simulink model "Filtro_pasa_bajo_2do_orden"  (R2023b)
settings: Solver=VariableStepAuto  StartTime=0.0  StopTime=10.0  RelTol=1e-3
undefined symbols (not defined in the file): wn, xita
settings Model: Creator=MSI  LastModifiedBy=MSI

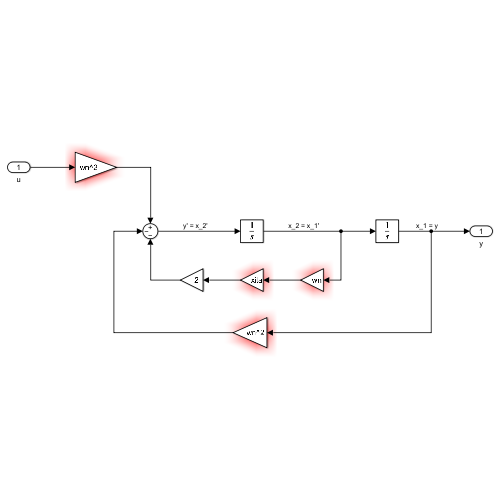
[thumbnail: Simulink's stored preview of the top-level diagram]
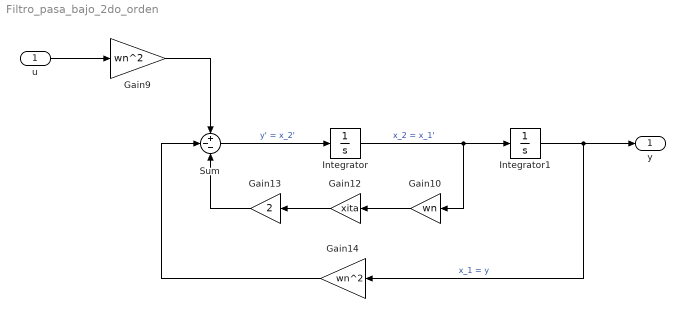
== system Filtro_pasa_bajo_2do_orden ==
  u : Inport
  Gain10 : Gain  Gain=wn
  Gain12 : Gain  Gain=xita
  Gain13 : Gain  Gain=2
  Gain14 : Gain  Gain=wn^2
  Gain9 : Gain  Gain=wn^2
  Integrator : Integrator
  Integrator1 : Integrator
  Sum : Sum  Inputs=+--
  y : Outport
  wires:
  Gain9/1 -> Sum/1
  Integrator1/1 -> Gain14/1, y/1  "x_1 = y"
  Gain10/1 -> Gain12/1
  Integrator/1 -> Gain10/1, Integrator1/1  "x_2 = x_1'"
  Gain12/1 -> Gain13/1
  Gain14/1 -> Sum/2
  Sum/1 -> Integrator/1  "y' = x_2'"
  Gain13/1 -> Sum/3
  u/1 -> Gain9/1
